simulink model "Final_Model"  (R2025b)
settings: Solver=ode4  StartTime=0.0  StopTime=5  FixedStep=0.01  RelTol=1e-3
libraries: arduinolib x4, slpidlib x1
settings Model: ExtModeTrigDuration=2  Creator=sid  LastModifiedBy=sid
settings SolverCC: AutoInsertRateTranBlk=on
settings OptimizationCC: EnhancedBackFolding=on  PassReuseOutputArgsAs=Individual arguments  ZeroExternalMemoryAtStartup=off  ZeroInternalMemoryAtStartup=off  MaxStackSize=64  OptimizeBlockOrder=speed  DifferentSizesBufferReuse=on  OptimizationCustomize=off  EfficientTunableParamExpr=on
settings DebuggingCC: MultiTaskDSMMsg=none  ParameterTunabilityLossMsg=error
settings HardwareCC: ProdBitPerPointer=32.0  ProdBitPerSizeT=32.0  ProdBitPerPtrDiffT=32.0  ProdLargestAtomicInteger=Long  ProdLargestAtomicFloat=Double  ProdWordSize=32.0  ProdHWDeviceType=ARM Compatible->ARM Cortex  UseEmbeddedCoderFeatures=off
settings SFSimCC: MATLABDynamicMemAlloc=off
settings RTWCC: SystemTargetFile=ert.tlc  HardwareBoard=ESP32-WROOM (Arduino Compatible)  TLCOptions="-aInlineSetEventsForThisBaseRateFcn=TLC_FALSE -aSuppressMultiTaskScheduler=TLC_FALSE  -aRateBasedStepFcn=0"  TemplateMakefile=ert_default_tmf  Toolchain=ESP32  Description=Embedded Coder
settings CodeAppCC: ForceParamTrailComments=on  IgnoreCustomStorageClasses=off  OperatorAnnotations=on  SimulinkDataObjDesc=on  SFDataObjDesc=on  InsertBlockDesc=on
settings ERTTargetCC: ExtModeTransport=3.0  ExtModeStaticAlloc=on  ExtModeAutomaticAllocSize=off  ExtModeStaticAllocSize=65536.0  ExtModeMexFile=ext_xcp  ExtModeIntrfLevel=Level2 - Open  InlinedParameterPlacement=Hierarchical  SupportContinuousTime=on  SupportNonInlinedSFcns=on  SupportVariableSizeSignals=on

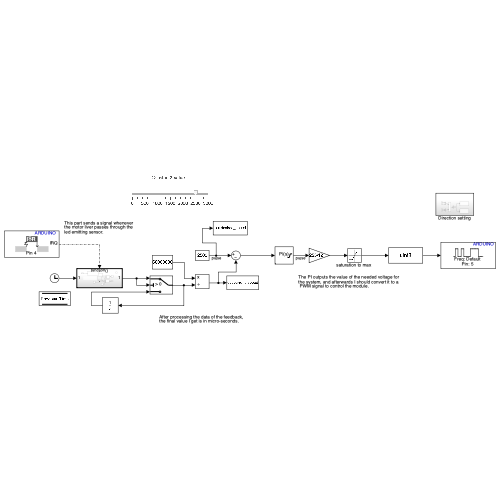
[thumbnail: Simulink's stored preview of the top-level diagram]
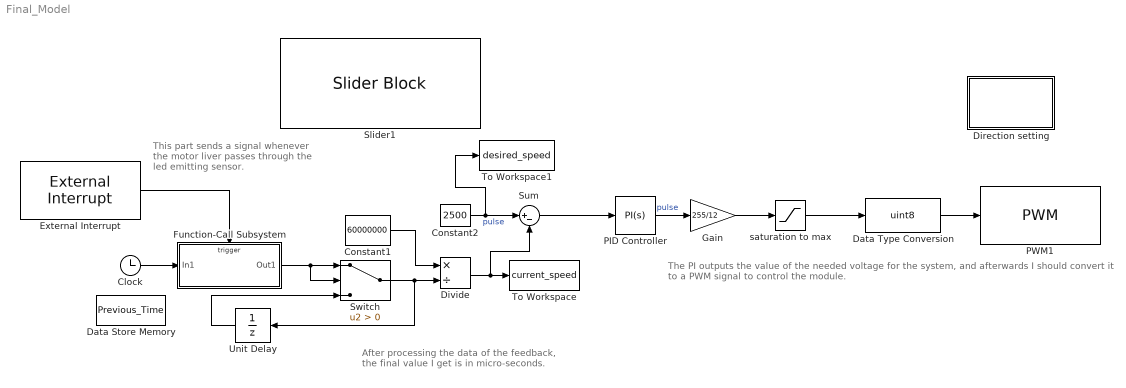
== system Final_Model ==
  note: After processing the data of the feedback,
      | the final value I get is in micro-seconds.
  note: The PI outputs the value of the needed voltage for
      | the system, and afterwards I should convert it to a
      |  PWM signal to control the module.
  note: This part sends a signal whenever
      | the motor liver passes through the
      | led emitting sensor.
  Clock : Clock
  Constant1 : Constant  Value=60000000
  Constant2 : Constant  Value=2500  OutMin=0  OutMax=3000
  Data Store Memory : DataStoreMemory  DataStoreName=Previous_Time  WriteAfterWriteMsg=warning  ShowAdditionalParam=off  OutDataTypeStr=uint32
  Data Type Conversion : DataTypeConversion  OutDataTypeStr=uint8  SaturateOnIntegerOverflow=off  RndMeth=Floor
  Direction setting : Subsystem
  Divide : Product  Inputs=*/
  External Interrupt : arduinolib/External Interrupt  Pin=4  PullUp=off  Mode=RISING  InterruptSimulationInput=off
  Function-Call Subsystem : Subsystem  TreatAsAtomicUnit=on
  Gain : Gain  Gain=255/12
  PID Controller : slpidlib/PID Controller  Controller=PI  Form=Parallel  TimeDomain=Continuous-time  UseExternalTs=off  SampleTime=-1  IntegratorMethod=Forward Euler  FilterMethod=Forward Euler  ControllerParametersSource=internal  P=0.00127586  I=0.01772978  UseKiTs=off  D=0  UseExternalDerivativeSource=off  N=100  UseFilter=on  TunerSelectOption=Transfer Function Based (PID Tuner App)  InitialConditionSource=internal  InitialConditionForIntegrator=0  InitialConditionForFilter=0  DifferentiatorICPrevScaledInput=0  ExternalReset=none  TrackingMode=off  Kt=1  LimitOutput=on  SatLimitsSource=internal  UpperSaturationLimit=12  LowerSaturationLimit=0  LinearizeAsGain=on  AntiWindupMode=none  Kb=1  LimitIntegrator=off  UpperIntegratorSaturationLimit=inf  LowerIntegratorSaturationLimit=-inf  POutMin=[]  POutMax=[]  IOutMin=[]  IOutMax=[]  DOutMin=[]  DOutMax=[]  NOutMin=[]  NOutMax=[]  SumOutMin=[]  SumOutMax=[]  SaturationOutMin=[]  SaturationOutMax=[]  PParamMin=[]  PParamMax=[]  IParamMin=[]  IParamMax=[]  DParamMin=[]  DParamMax=[]  NParamMin=[]  NParamMax=[]  KbParamMin=[]  KbParamMax=[]  KtParamMin=[]  KtParamMax=[]  KbOutMin=[]  KbOutMax=[]  KtOutMin=[]  KtOutMax=[]  IntegratorOutMin=[]  IntegratorOutMax=[]  FilterOutMin=[]  FilterOutMax=[]  SumI1OutMin=[]  SumI1OutMax=[]  SumI2OutMin=[]  SumI2OutMax=[]  SumI3OutMin=[]  SumI3OutMax=[]  SumI4OutMin=[]  SumI4OutMax=[]  SumDOutMin=[]  SumDOutMax=[]  DifferentiatorOutMin=[]  DifferentiatorOutMax=[]  FilterDiffOutCoefMin=[]  FilterDiffOutCoefMax=[]  ReciprocalOutMin=[]  ReciprocalOutMax=[]  SumDenOutMin=[]  SumDenOutMax=[]  SumNumOutMin=[]  SumNumOutMax=[]  DivideOutMin=[]  DivideOutMax=[]  UdiffTsProdOutMin=[]  UdiffTsProdOutMax=[]  NTsProdOutMin=[]  NTsProdOutMax=[]  UintegralTsProdOutMin=[]  UintegralTsProdOutMax=[]  UngainTsProdOutMin=[]  UngainTsProdOutMax=[]  ClampingZeroOutDataTypeStr=Inherit: Inherit via back propagation  ClampingZeroOutMin=[]  ClampingZeroOutMax=[]  FilterDenConstantOutDataTypeStr=Inherit: Inherit via back propagation  FilterDenConstantOutMin=[]  FilterDenConstantOutMax=[]  PCopyOutDataTypeStr=Inherit: Inherit via back propagation  PCopyOutMin=[]  PCopyOutMax=[]  NCopyOutDataTypeStr=Inherit: Inherit via back propagation  NCopyOutMin=[]  NCopyOutMax=[]  IntegratorContinuousStateAttributes=''  IntegratorStateMustResolveToSignalObject=off  IntegratorRTWStateStorageClass=Auto  FilterContinuousStateAttributes=''  FilterStateMustResolveToSignalObject=off  FilterRTWStateStorageClass=Auto  ParallelPVariant=InternalParameters  IdealPVariant=Disabled  IVariant=InternalParameters  DVariant=Disabled  IntegratorVariant=Continuous  SatVariant=Enabled  AWVariant=Passthrough  PCopyVariant=Disabled  TRVariant=Disabled  FdbkBlocksVariant=Forward  IdealPFdbkVariant=Disabled  SatFdbkVariant=Disabled  DerivativeFilterVariant=Disabled  NVariant=Disabled  NCopyVariant=Disabled_SignalSpec  FilterICVariant=Disabled  IntegratorICVariant=InternalICs  ExternalResetVariant=Disabled  TRSumVariant=Passthrough  SumFdbkVariant=Disabled  SumVariant=Sum_PI  TsampFilterVariant=InternalTs  TsampNgainVariant=Passthrough  TsampIntegralVariant=Disabled_SignalSpec  ExternalSaturationOutDataTypeStr=Inherit: Same as second input  DerivativeSourceVariant=Disabled  PreIntVariant=InternalPreInt
  PWM1 : arduinolib/PWM  pinNumber=5  frequencyType=Default  desiredFrequency=490.2  achievableFrequency=490.2
  Slider1 : SliderBlock  ScaleMax=3000
  Sum : Sum  Inputs=|+-
  Switch : Switch  Criteria=u2 > Threshold  SaturateOnIntegerOverflow=off  InputSameDT=off
  To Workspace : ToWorkspace  VariableName=current_speed  SaveFormat=Timeseries  SampleTime=-1
  To Workspace1 : ToWorkspace  VariableName=desired_speed  SaveFormat=Timeseries  SampleTime=-1
  Unit Delay : UnitDelay  InitialCondition=60000000  SampleTime=-1  HasFrameUpgradeWarning=on
  "saturation to max " : Saturate  UpperLimit=255  LowerLimit=0
  wires:
  Data Type Conversion/1 -> PWM1/1
  "saturation to max "/1 -> Data Type Conversion/1
  Gain/1 -> "saturation to max "/1
  Divide/1 -> To Workspace/1, Sum/2
  Constant2/1 -> To Workspace1/1, Sum/1  "pulse"
  Switch/1 -> Divide/2, Unit Delay/1
  Unit Delay/1 -> Switch/3
  PID Controller/1 -> Gain/1  "pulse"
  Function-Call Subsystem/1(Out1) -> Switch/2, Switch/1
  Sum/1 -> PID Controller/1
  Clock/1 -> Function-Call Subsystem/1(In1)
  Constant1/1 -> Divide/1
  External Interrupt/1 -> Function-Call Subsystem/Trigger

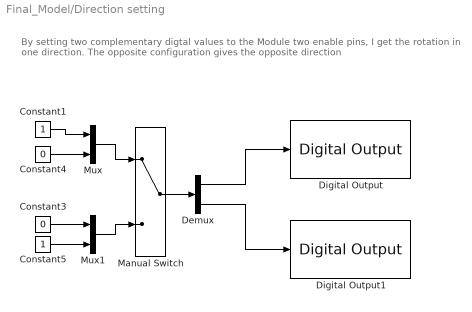
== system Final_Model/Direction setting ==
  note: By setting two complementary digtal values to the Module two enable pins, I get the rotation in one direction. The opposite configuration gives the opposite direction
  Constant1 : Constant  OutMin=0  OutMax=1  OutDataTypeStr=uint8
  Constant3 : Constant  Value=0  OutMin=0  OutMax=1  OutDataTypeStr=uint8
  Constant4 : Constant  Value=0  OutMin=0  OutMax=1  OutDataTypeStr=uint8
  Constant5 : Constant  OutMin=0  OutMax=1  OutDataTypeStr=uint8
  Demux : Demux  Outputs=2
  Digital Output : arduinolib/Digital Output  pinNumber=19  Direction=output  blockPlatform=arduino
  Digital Output1 : arduinolib/Digital Output  pinNumber=21  Direction=output  blockPlatform=arduino
  Manual Switch : ManualSwitch
  Mux : Mux  Inputs=2
  Mux1 : Mux  Inputs=2
  wires:
  Constant4/1 -> Mux/2
  Mux1/1 -> Manual Switch/2
  Demux/1 -> Digital Output/1
  Demux/2 -> Digital Output1/1
  Constant1/1 -> Mux/1
  Mux/1 -> Manual Switch/1
  Constant5/1 -> Mux1/2
  Constant3/1 -> Mux1/1
  Manual Switch/1 -> Demux/1

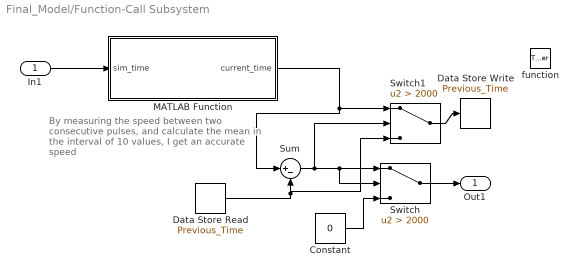
== system Final_Model/Function-Call Subsystem ==
  note: By measuring the speed between
      | two consecutive pulses,
      | and calculate the mean in the
      | interval of 10 values, I get an accurate speed
  In1 : Inport
  function : TriggerPort  TriggerType=function-call  VariantControl=(inherit)
  Constant : Constant  Value=0
  Data Store Read : DataStoreRead  Priority=1  DataStoreName=Previous_Time  IndexOptions=Index vector (dialog)  Indices=1  OutputSizes=1
  Data Store Write : DataStoreWrite  Priority=10  DataStoreName=Previous_Time  IndexOptions=Index vector (dialog)  Indices=1  OutputSizes=1
  MATLAB Function : MATLAB Function  TreatAsAtomicUnit=on
  Sum : Sum  Inputs=|+-
  Switch : Switch  Criteria=u2 > Threshold  Threshold=2000  SaturateOnIntegerOverflow=off  InputSameDT=off
  Switch1 : Switch  Criteria=u2 > Threshold  Threshold=2000  SaturateOnIntegerOverflow=off  InputSameDT=off
  Out1 : Outport
  wires:
  Data Store Read/1 -> Switch1/3, Sum/2
  MATLAB Function/1(current_time) -> Switch1/1, Sum/1
  In1/1 -> MATLAB Function/1(sim_time)
  Sum/1 -> Switch1/2, Switch/2, Switch/1
  Switch/1 -> Out1/1
  Constant/1 -> Switch/3
  Switch1/1 -> Data Store Write/1

== matlab function Final_Model/Function-Call Subsystem/MATLAB Function ==
  data: current_time output; sim_time input
function current_time = get_micros(sim_time)
    current_time = uint32(0); 
    
    if coder.target('rtw')
        % --- HARDWARE MODE (ESP32) ---
        % Call the C function 'micros()' directly
        current_time = coder.ceval('micros'); 
        
    else
        % --- SIMULATION MODE (Computer) ---
        % Convert the Simulation Time (seconds) to Microseconds
        % 1 second = 1,000,000 microseconds
        current_time = uint32(sim_time * 1000000);
    end
end
